simulink model "inverter_3p3s"  (R2018a)
settings: Solver=FixedStepDiscrete  StartTime=0.0  StopTime=stop_time  FixedStep=step_size  RelTol=1e-3
InitFcn:
  | param
values from neighbouring files (symbols this model uses):
  C_DC = 100e-6    (= 0.0001)    [param.m]
  C_DC_ESL = 1e-6    (= 1e-06)    [param.m]
  C_DC_ESR = 1e-1    (= 0.1)    [param.m]
  CpA = 10e-9    (= 1e-08)    [param.m]
  CpB = 12e-9    (= 1.2e-08)    [param.m]
  CpC = 10e-9    (= 1e-08)    [param.m]
  duty = 0.5    [param.m]
  f_resonance = 1/(2*pi*sqrt(LpA*CpA))    [param.m]
  L_DC = 1e-6    (= 1e-06)    [param.m]
  LpA = 80e-6    (= 8e-05)    [param.m]
  LpB = 50e-6    (= 5e-05)    [param.m]
  LpC = 67e-6    (= 6.7e-05)    [param.m]
  R_DC = 1e-1    (= 0.1)    [param.m]
  RpA = 12    [param.m]
  RpB = 6    [param.m]
  RpC = 10    [param.m]
  step_size = 1e-9    (= 1e-09)    [param.m]
  V_DC = 100    [param.m]
libraries: powerlib x18
settings Model: Creator=enes_  LastModifiedBy=enes_

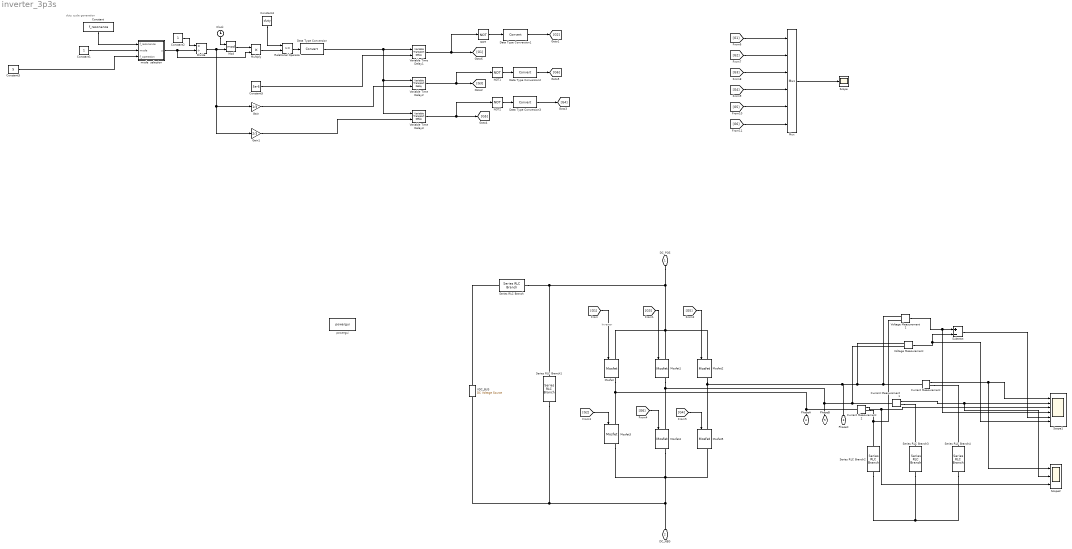
== system inverter_3p3s ==
  note: duty cycle generation
  note: Inverter
  Clock : Clock
  Constant : Constant  Value=f_resonance
  Constant1 : Constant
  Constant2 : Constant
  Constant3 : Constant  Value=5
  Constant4 : Constant  Value=duty
  Constant5 : Constant  Value=5e-6
  Current Measurement : powerlib/Measurements/Current Measurement  PhasorSimulation=off  OutputType=Complex  PSBequivalent=0
  Current Measurement1 : powerlib/Measurements/Current Measurement  PhasorSimulation=off  OutputType=Complex  PSBequivalent=0
  Current Measurement2 : powerlib/Measurements/Current Measurement  PhasorSimulation=off  OutputType=Complex  PSBequivalent=0
  Data Type Conversion{,1..3} (4 alike) : DataTypeConversion
  Divide : Product  Inputs=*/
  Gain : Gain  Gain=1/3
  Gain1 : Gain  Gain=2/3
  Mod : Math  Operator=mod  SaturateOnIntegerOverflow=on
  Mosfet{,1..5} (6 alike) : powerlib/Power Electronics/Mosfet  Ron=0.1  Lon=0  Rd=0.01  Vfd=0  IC=0  Rs=1e5  Cs=inf  Measurements=on
  Multiply : Product
  Mux : Mux  Inputs=6
  NOT : Logic  Operator=NOT  IconShape=distinctive  AllPortsSameDT=off  OutDataTypeStr=boolean
  NOT1 : Logic  Operator=NOT  IconShape=distinctive  AllPortsSameDT=off  OutDataTypeStr=boolean
  NOT2 : Logic  Operator=NOT  IconShape=distinctive  AllPortsSameDT=off  OutDataTypeStr=boolean
  Relational Operator : RelationalOperator  OutDataTypeStr=boolean  RndMeth=Simplest
  Scope : Scope
  Scope1 : Scope  NumInputPorts=6
  Scope2 : Scope  NumInputPorts=3
  Series RLC Branch : powerlib/Elements/Series RLC Branch  LConnTagsString=__new0  RConnTagsString=__new0  BranchType=RL  Resistance=R_DC  Inductance=L_DC  SetiL0=off  InitialCurrent=0  Capacitance=1e-6  Setx0=off  InitialVoltage=0  Measurements=None
  Series RLC Branch1 : powerlib/Elements/Series RLC Branch  LConnTagsString=__new0  RConnTagsString=__new0  BranchType=RLC  Resistance=C_DC_ESR  Inductance=C_DC_ESL  SetiL0=off  InitialCurrent=0  Capacitance=C_DC  Setx0=off  InitialVoltage=0  Measurements=None
  Series RLC Branch2 : powerlib/Elements/Series RLC Branch  LConnTagsString=__new0  RConnTagsString=__new0  BranchType=RLC  Resistance=RpA  Inductance=LpA  SetiL0=off  InitialCurrent=0  Capacitance=CpA  Setx0=off  InitialVoltage=0  Measurements=None
  Series RLC Branch3 : powerlib/Elements/Series RLC Branch  LConnTagsString=__new0  RConnTagsString=__new0  BranchType=RLC  Resistance=RpB  Inductance=LpB  SetiL0=off  InitialCurrent=0  Capacitance=CpB  Setx0=off  InitialVoltage=0  Measurements=None
  Series RLC Branch4 : powerlib/Elements/Series RLC Branch  LConnTagsString=__new0  RConnTagsString=__new0  BranchType=RLC  Resistance=RpC  Inductance=LpC  SetiL0=off  InitialCurrent=0  Capacitance=CpC  Setx0=off  InitialVoltage=0  Measurements=None
  Subtract : Sum  Inputs=+-
  VDC_BUS : powerlib/Electrical Sources/DC Voltage Source  Amplitude=V_DC  Measurements=None
  Variable Time Delay1 : VariableTransportDelay  MaximumDelay=10
  Variable Time Delay2 : VariableTransportDelay  MaximumDelay=10
  Variable Time Delay3 : VariableTransportDelay  MaximumDelay=10
  Voltage Measurement : powerlib/Measurements/Voltage Measurement  PhasorSimulation=off  OutputType=Complex  PSBequivalent=0
  Voltage Measurement1 : powerlib/Measurements/Voltage Measurement  PhasorSimulation=off  OutputType=Complex  PSBequivalent=0
  mode  selection : MATLAB Function  TreatAsAtomicUnit=on
  powergui : powerlib/powergui  Priority=1  SimulationMode=Discrete  SampleTime=step_size  frequency=60  Iterations=50  frequencyindice=0  Pbase=100e6  ErrMax=1e-4  UnitsV=kV  UnitsW=MW  buscounter=0  FunctionMessages=off  echomessages=off  EnableUseOfTLC=off  CurrentSourceSwitches=off  DisableSnubberDevices=off  DisableRonSwitches=off  DisableVfSwitches=off  DisplayEquations=off  SolverType=Tustin/Backward Euler (TBE)  Interpol=off  ExternalGateDelay=off  methode=off  Ts=100  x0status=blocks  SPID=on  SwTol=0  HookPort=off  RestoreLinks=warning  ResistiveCurrentMeasurement=off  Frange=[0:2:500]  Ylog=off  Xlog=on  ShowGrid=off  save=off  variable=ZData  structure=0  ZoomFFT=off  StartTime=0.0  cycles=1  DisplayStyle=1  fundamental=60  FreqAxis=off  MaxFrequency=1000  frequencyindicesteady=1  RmsSteady=1  display=off
  DC_POS : PMIOPort  Side=Left
  DC_NEG : PMIOPort  Port=2  Side=Left
  PhaseC : PMIOPort  Port=3  Side=Left
  PhaseA : PMIOPort  Port=4  Side=Left
  PhaseB : PMIOPort  Port=5  Side=Left
  wires:
  [G5] -> Mosfet2/1
  Constant2/1 -> Divide/1
  Clock/1 -> Mod/1
  Constant/1 -> mode  selection/1(f_resonance)
  Constant1/1 -> mode  selection/2(mode)
  Relational Operator/1 -> Data Type Conversion/1
  mode  selection/1(y) -> Multiply/2, Divide/2
  Constant3/1 -> mode  selection/3(f_operation)
  Constant4/1 -> Relational Operator/1
  Multiply/1 -> Relational Operator/2
  Data Type Conversion/1 -> Variable Time Delay3/1, Variable Time Delay2/1, Variable Time Delay1/1
  Divide/1 -> Gain1/1, Gain/1, Mod/2
  Mod/1 -> Multiply/1
  Variable Time Delay1/1 -> NOT/1, [G1]
  [G1] -> Mosfet/1
  Variable Time Delay2/1 -> NOT1/1, [G3]
  [G3] -> Mosfet1/1
  Constant5/1 -> Variable Time Delay1/2
  Gain1/1 -> Variable Time Delay3/2
  NOT/1 -> Data Type Conversion1/1
  NOT1/1 -> Data Type Conversion2/1
  Data Type Conversion1/1 -> [G2]
  Data Type Conversion2/1 -> [G6]
  NOT2/1 -> Data Type Conversion3/1
  Data Type Conversion3/1 -> [G4]
  Variable Time Delay3/1 -> NOT2/1, [G5]
  [G2] -> Mosfet3/1
  [G6] -> Mosfet4/1
  [G4] -> Mosfet5/1
  [G1] -> Mux/1
  [G2] -> Mux/2
  [G3] -> Mux/3
  [G4] -> Mux/4
  [G5] -> Mux/5
  [G6] -> Mux/6
  Mux/1 -> Scope/1
  Current Measurement/1 -> Scope2/1, Scope1/1
  Current Measurement1/1 -> Scope2/2, Scope1/2
  Current Measurement2/1 -> Scope2/3, Scope1/3
  Voltage Measurement1/1 -> Scope1/4, Subtract/1
  Voltage Measurement/1 -> Scope1/6, Subtract/2
  Subtract/1 -> Scope1/5
  Gain/1 -> Variable Time Delay2/2
  connections:
  Mosfet/RConn1 -- Current Measurement2/LConn1 -- PhaseA/RConn1 -- Mosfet3/LConn1
  Mosfet1/RConn1 -- Voltage Measurement/LConn2 -- Current Measurement1/LConn1 -- PhaseB/RConn1 -- Mosfet4/LConn1
  Mosfet/LConn1 -- Series RLC Branch1/LConn1 -- Series RLC Branch/RConn1 -- DC_POS/RConn1 -- Mosfet1/LConn1 -- Mosfet2/LConn1
  Mosfet3/RConn1 -- VDC_BUS/LConn1 -- Series RLC Branch1/RConn1 -- DC_NEG/RConn1 -- Mosfet4/RConn1 -- Mosfet5/RConn1
  VDC_BUS/RConn1 -- Series RLC Branch/LConn1
  Series RLC Branch2/RConn1 -- Series RLC Branch4/RConn1 -- Series RLC Branch3/RConn1
  Current Measurement/RConn1 -- Series RLC Branch4/LConn1
  Current Measurement1/RConn1 -- Series RLC Branch3/LConn1
  Mosfet2/RConn1 -- Voltage Measurement1/LConn1 -- Current Measurement/LConn1 -- Voltage Measurement/LConn1 -- PhaseC/RConn1 -- Mosfet5/LConn1
  Current Measurement2/RConn1 -- Voltage Measurement1/LConn2 -- Series RLC Branch2/LConn1

== matlab function inverter_3p3s/mode  selection ==
  data: f_resonance input; y output; mode input; f_operation input
function y = fcn(f_resonance, mode, f_operation)

if mode ==0 
    y = f_operation;
    
else 
    y=f_resonance;
    
end
